simulink model "simulink_priklad"  (R2017b)
settings: Solver=VariableStepAuto  StartTime=0.0  StopTime=10.0  RelTol=1e-3
settings Model: Creator=nanom  LastModifiedBy=nanom

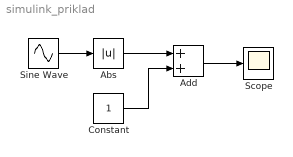
== system simulink_priklad ==
  Abs : Abs
  Add : Sum
  Constant : Constant
  Scope : Scope
  Sine Wave : Sin  SampleTime=0
  wires:
  Sine Wave/1 -> Abs/1
  Abs/1 -> Add/1
  Add/1 -> Scope/1
  Constant/1 -> Add/2
